simulink model "exemples_subscriber"  (R2018a)
settings: Solver=VariableStepAuto  StartTime=0.0  StopTime=10.0  RelTol=1e-3
libraries: robotlib x3
settings Model: Creator=root  LastModifiedBy=root

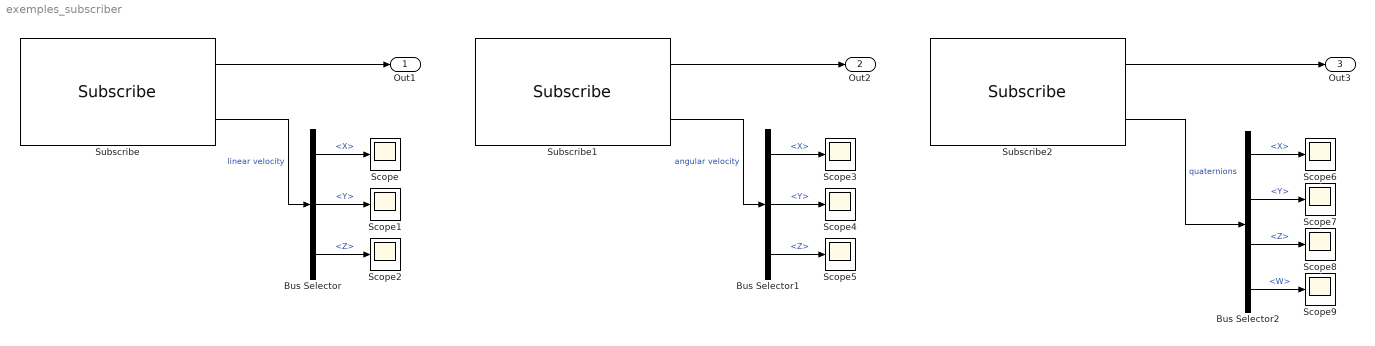
== system exemples_subscriber ==
  Bus Selector : BusSelector  OutputSignals=Twist.Linear.X,Twist.Linear.Y,Twist.Linear.Z
  Bus Selector1 : BusSelector  OutputSignals=Twist.Angular.X,Twist.Angular.Y,Twist.Angular.Z
  Bus Selector2 : BusSelector  OutputSignals=Pose.Orientation.X,Pose.Orientation.Y,Pose.Orientation.Z,Pose.Orientation.W
  Scope{,1..9} (10 alike) : Scope
  Subscribe : robotlib/Subscribe  SourceLibraryInfo=This block requires Robotics System Toolbox  topicSource=Select from ROS network  topic=/ual/velocity  messageType=geometry_msgs/TwistStamped  sampleTime=inf  messageQueueLength=1
      settings: SourceProductBaseCode=RO
  Subscribe1 : robotlib/Subscribe  SourceLibraryInfo=This block requires Robotics System Toolbox  topicSource=Select from ROS network  topic=/ual/set_velocity  messageType=geometry_msgs/TwistStamped  sampleTime=inf  messageQueueLength=1
      settings: SourceProductBaseCode=RO
  Subscribe2 : robotlib/Subscribe  SourceLibraryInfo=This block requires Robotics System Toolbox  topicSource=Select from ROS network  topic=/ual/pose  messageType=geometry_msgs/PoseStamped  sampleTime=inf  messageQueueLength=1
      settings: SourceProductBaseCode=RO
  Out1 : Outport
  Out2 : Outport  Port=2
  Out3 : Outport  Port=3
  wires:
  Subscribe/2 -> Bus Selector/1  "linear velocity"
  Bus Selector/1 -> Scope/1  "<X>"
  Bus Selector/2 -> Scope1/1  "<Y>"
  Bus Selector/3 -> Scope2/1  "<Z>"
  Subscribe/1 -> Out1/1
  Bus Selector1/2 -> Scope4/1  "<Y>"
  Bus Selector1/3 -> Scope5/1  "<Z>"
  Bus Selector1/1 -> Scope3/1  "<X>"
  Subscribe1/2 -> Bus Selector1/1  "angular velocity"
  Subscribe1/1 -> Out2/1
  Bus Selector2/3 -> Scope8/1  "<Z>"
  Bus Selector2/2 -> Scope7/1  "<Y>"
  Bus Selector2/1 -> Scope6/1  "<X>"
  Subscribe2/1 -> Out3/1
  Subscribe2/2 -> Bus Selector2/1  "quaternions"
  Bus Selector2/4 -> Scope9/1  "<W>"
